simulink model "division"  (R2022b)
settings: Solver=FixedStepDiscrete  StartTime=0.0  StopTime=0.0002  RelTol=1e-3
model workspace (MAT data in the model file):
  test = 0
libraries: hdlsllib x4
settings Model: DataTypeOverride=Off  FPTShortcutValueString='{{},{''BaselineRun'',1,1,1,''BaselineRun'','''',{},''M'',''F'',''''},{''EmbeddedRun'',1,1,1,''EmbeddedRun'','''',{},''M'','''',''''}}'  Creator=max_d  LastModifiedBy=bennizette
settings SolverCC: AlgebraicLoopSolver=TrustRegion  AutoInsertRateTranBlk=on
settings DataIOCC: LimitDataPoints=on  SaveOutput=off  SaveTime=off
settings OptimizationCC: BlockReduction=off  ConditionallyExecuteInputs=off  DefaultParameterBehavior=Inlined  InheritOutputTypeSmallerThanSingle=on  LifeSpan=inf
settings DebuggingCC: SignalRangeChecking=warning  AlgebraicLoopMsg=error  SingleTaskRateTransMsg=error  UnconnectedInputMsg=warning  UnconnectedOutputMsg=warning  UnconnectedLineMsg=warning  AllowSymbolicDim=off  StrictBusMsg=ErrorOnBusTreatedAsVector  SFUnexpectedBacktrackingDiag=warning  SFNoUnconditionalDefaultTransitionDiag=warning  SFExecutionAtInitializationDiag=none  SFMachineParentedDataDiag=warning  ArithmeticOperatorsInVariantConditions=warning
settings HardwareCC: ProdBitPerPointer=32  ProdBitPerSizeT=32  ProdBitPerPtrDiffT=32  ProdLargestAtomicFloat=None  ProdIntDivRoundTo=Undefined  ProdEndianess=Unspecified  ProdWordSize=32  ProdHWDeviceType=ASIC/FPGA->ASIC/FPGA  ProdEqTarget=off
settings ModelReferenceCC: EnableRefExpFcnMdlSchedulingChecks=on
settings SFSimCC: SimUseLocalCustomCode=off  CustomCodeUndefinedFunction=UseInterfaceOnly
settings RTWCC: RTWUseLocalCustomCode=off  DLArmComputeVersion=19.05
settings CodeAppCC: StateflowObjectComments=on
settings GRTTargetCC: TargetLangStandard=C89/C90 (ANSI)
settings ConfigComp: CovScope=ReferencedModels  CovMetricSettings=dw  CovSaveCumulativeToWorkspaceVar=on  CovSaveSingleToWorkspaceVar=on  CovExternalEMLEnable=off  CovSFcnEnable=off

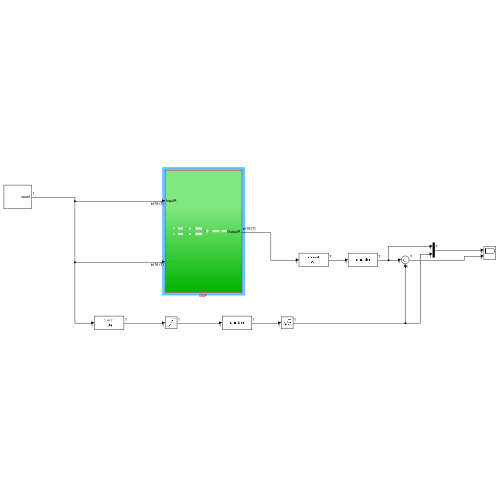
[thumbnail: Simulink's stored preview of the top-level diagram]
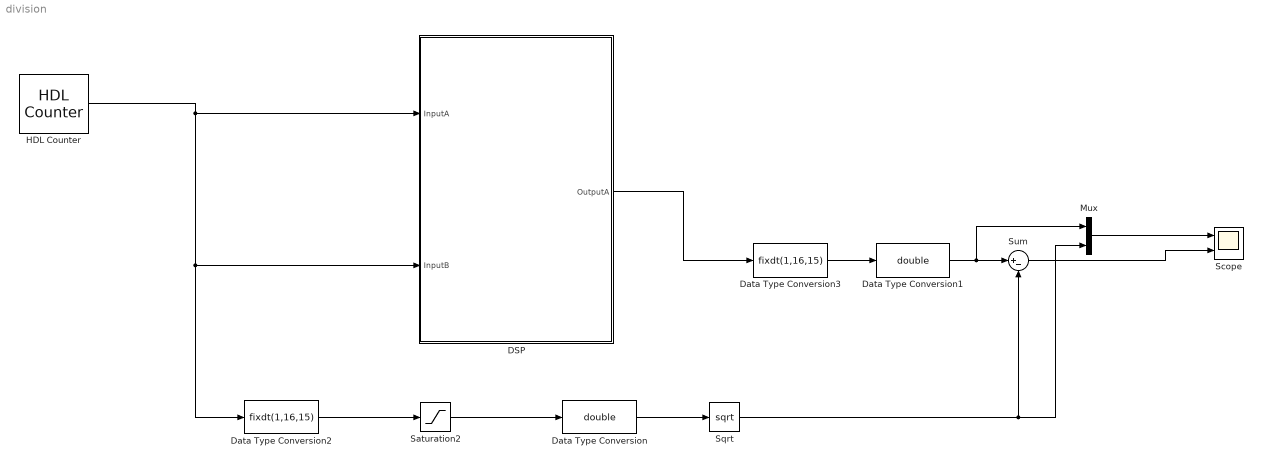
== system division ==
  DSP : Subsystem
  Data Type Conversion : DataTypeConversion  OutDataTypeStr=double  SaturateOnIntegerOverflow=off  RndMeth=Floor
  Data Type Conversion1 : DataTypeConversion  OutDataTypeStr=double  SaturateOnIntegerOverflow=off  RndMeth=Floor
  Data Type Conversion2 : DataTypeConversion  OutDataTypeStr=fixdt(1,16,15)  ConvertRealWorld=Stored Integer (SI)  SaturateOnIntegerOverflow=off  RndMeth=Floor
  Data Type Conversion3 : DataTypeConversion  OutDataTypeStr=fixdt(1,16,15)  ConvertRealWorld=Stored Integer (SI)  SaturateOnIntegerOverflow=off  RndMeth=Floor
  HDL Counter : hdlsllib/Sources/HDL Counter  CountType=Free running  CountInit=0  CountStep=1  CountMax=25  CountFromType=Initial value  CountFrom=0  CountResetPort=off  CountLoadPort=off  CountEnbPort=off  CountDirPort=off  CountHitOutputPort=off  CountDataType=Signed  CountWordLen=16  CountFracLen=0  CountSampTime=1/312.5e6
  Mux : Mux  Inputs=2
  Saturation2 : Saturate  UpperLimit=1  LowerLimit=0
  Scope : Scope  NumInputPorts=2
  Sqrt : Sqrt
  Sum : Sum  Inputs=|+-
  wires:
  HDL Counter/1 -> Data Type Conversion2/1, DSP/2(InputB), DSP/1(InputA)
  Sqrt/1 -> Mux/2, Sum/2
  Data Type Conversion1/1 -> Mux/1, Sum/1
  Saturation2/1 -> Data Type Conversion/1
  Data Type Conversion/1 -> Sqrt/1
  Data Type Conversion2/1 -> Saturation2/1
  DSP/1(OutputA) -> Data Type Conversion3/1
  Data Type Conversion3/1 -> Data Type Conversion1/1
  Mux/1 -> Scope/1
  Sum/1 -> Scope/2

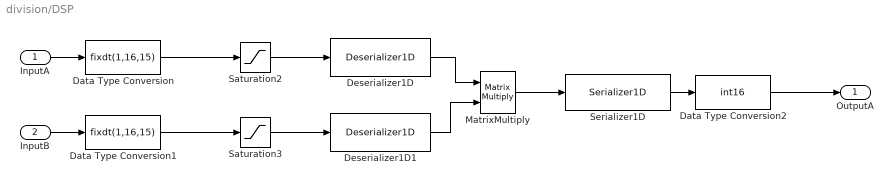
== system division/DSP ==
  InputA : Inport  OutDataTypeStr=fixdt(1,16,0)
  InputB : Inport  Port=2  OutDataTypeStr=fixdt(1,16,0)
  Data Type Conversion : DataTypeConversion  OutDataTypeStr=fixdt(1,16,15)  ConvertRealWorld=Stored Integer (SI)  SaturateOnIntegerOverflow=off  RndMeth=Floor
  Data Type Conversion1 : DataTypeConversion  OutDataTypeStr=fixdt(1,16,15)  ConvertRealWorld=Stored Integer (SI)  SaturateOnIntegerOverflow=off  RndMeth=Floor
  Data Type Conversion2 : DataTypeConversion  OutDataTypeStr=int16  ConvertRealWorld=Stored Integer (SI)  SaturateOnIntegerOverflow=off  RndMeth=Floor
  Deserializer1D : hdlsllib/HDL Operations/Deserializer1D  Ratio=100  IdleCycles=0  InitialCondition=0  startIn=off  validIn=off  validOut=off  inputDataDimensions=-1  inputSampleTime=-1  inputSignalType=auto
  Deserializer1D1 : hdlsllib/HDL Operations/Deserializer1D  Ratio=100  IdleCycles=0  InitialCondition=0  startIn=off  validIn=off  validOut=off  inputDataDimensions=-1  inputSampleTime=-1  inputSignalType=auto
  MatrixMultiply : Product  Multiplication=Matrix(*)
  Saturation2 : Saturate  UpperLimit=1  LowerLimit=0
  Saturation3 : Saturate  UpperLimit=1  LowerLimit=0
  Serializer1D : hdlsllib/HDL Operations/Serializer1D  Ratio=100  IdleCycles=0  validIn=off  startOut=off  validOut=off  inputDataDimensions=-1  inputSampleTime=-1  inputSignalType=auto
  OutputA : Outport  OutDataTypeStr=fixdt(1,16,0)  VectorParamsAs1DForOutWhenUnconnected=off
  wires:
  InputA/1 -> Data Type Conversion/1
  InputB/1 -> Data Type Conversion1/1
  Serializer1D/1 -> Data Type Conversion2/1
  Data Type Conversion2/1 -> OutputA/1
  Data Type Conversion/1 -> Saturation2/1
  Data Type Conversion1/1 -> Saturation3/1
  Saturation2/1 -> Deserializer1D/1
  Saturation3/1 -> Deserializer1D1/1
  Deserializer1D/1 -> MatrixMultiply/1
  Deserializer1D1/1 -> MatrixMultiply/2
  MatrixMultiply/1 -> Serializer1D/1
